simulink model "sensor"  (R2021a)
settings: Solver=VariableStepAuto  StartTime=0.0  StopTime=10.0  RelTol=1e-3
settings Model: Creator=may9c  LastModifiedBy=may9c

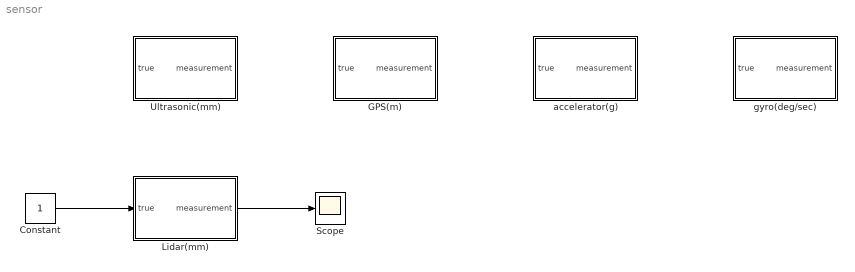
== system sensor ==
  Constant : Constant
  GPS(m) : Subsystem
  Lidar(mm) : Subsystem
  Scope : Scope
  Ultrasonic(mm) : Subsystem
  accelerator(g) : Subsystem
  gyro(deg/sec) : Subsystem
  wires:
  Constant/1 -> Lidar(mm)/1(true)
  Lidar(mm)/1(measurement) -> Scope/1

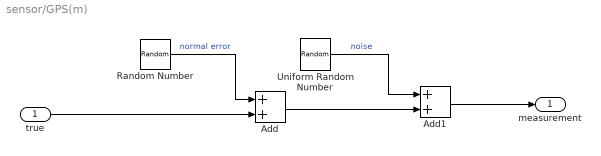
== system sensor/GPS(m) ==
  true : Inport
  Add : Sum
  Add1 : Sum
  Random Number : RandomNumber  Variance=2566.289833  SampleTime=0.1
  Uniform Random Number : UniformRandomNumber  SampleTime=0.1
  measurement : Outport
  wires:
  Add1/1 -> measurement/1
  Random Number/1 -> Add/1  "normal error"
  Uniform Random Number/1 -> Add1/1  "noise"
  Add/1 -> Add1/2
  true/1 -> Add/2

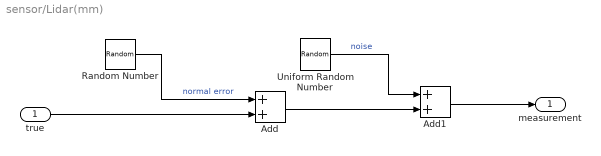
== system sensor/Lidar(mm) ==
  true : Inport
  Add : Sum
  Add1 : Sum
  Random Number : RandomNumber  Variance=41060.63732  SampleTime=0.1
  Uniform Random Number : UniformRandomNumber  SampleTime=0.1
  measurement : Outport
  wires:
  Add1/1 -> measurement/1
  Random Number/1 -> Add/1  "normal error"
  Uniform Random Number/1 -> Add1/1  "noise"
  Add/1 -> Add1/2
  true/1 -> Add/2

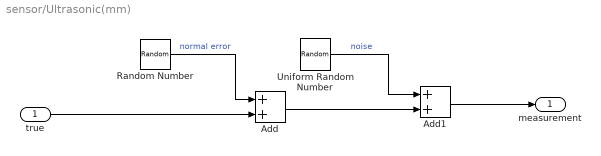
== system sensor/Ultrasonic(mm) ==
  true : Inport
  Add : Sum
  Add1 : Sum
  Random Number : RandomNumber  Variance=577415.2124  SampleTime=0.1
  Uniform Random Number : UniformRandomNumber  SampleTime=0.1
  measurement : Outport
  wires:
  Add1/1 -> measurement/1
  Random Number/1 -> Add/1  "normal error"
  Uniform Random Number/1 -> Add1/1  "noise"
  Add/1 -> Add1/2
  true/1 -> Add/2

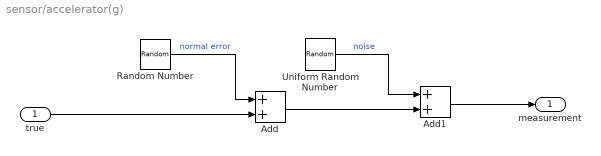
== system sensor/accelerator(g) ==
  true : Inport
  Add : Sum
  Add1 : Sum
  Random Number : RandomNumber  Variance=410.6064  SampleTime=0.1
  Uniform Random Number : UniformRandomNumber  SampleTime=0.1
  measurement : Outport
  wires:
  Add1/1 -> measurement/1
  Random Number/1 -> Add/1  "normal error"
  Uniform Random Number/1 -> Add1/1  "noise"
  Add/1 -> Add1/2
  true/1 -> Add/2

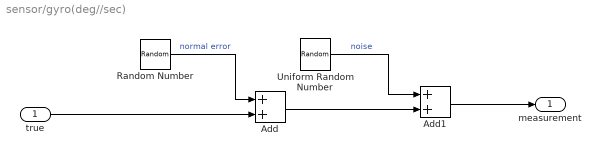
== system sensor/gyro(deg//sec) ==
  true : Inport
  Add : Sum
  Add1 : Sum
  Random Number : RandomNumber  Variance=1603931.145  SampleTime=0.1
  Uniform Random Number : UniformRandomNumber  SampleTime=0.1
  measurement : Outport
  wires:
  Add1/1 -> measurement/1
  Random Number/1 -> Add/1  "normal error"
  Uniform Random Number/1 -> Add1/1  "noise"
  Add/1 -> Add1/2
  true/1 -> Add/2
